simulink library "LibEEPROM_eeprom_example_ORIGINAL"  (Simulink 10.0)
settings: Solver=VariableStepAuto  StartTime=0.0  StopTime=10.0  RelTol=1e-3
undefined symbols (not defined in the file): CRC32_calc_and_EEPROM_Write_ALL, crc32_calc_intern, CRC32_EEPROM_Read, EEPROM_Mirror, EEPROM_Read, IO_Blk_Lib_TTC500, IO_EEPROM_GetStatus, IO_EEPROM_Init, IO_EEPROM_Write, Read_Mirror, Write_Mirror, Write_Mirror_prepare_EEPROM
libraries: simulink x56
(part 3 of 8)

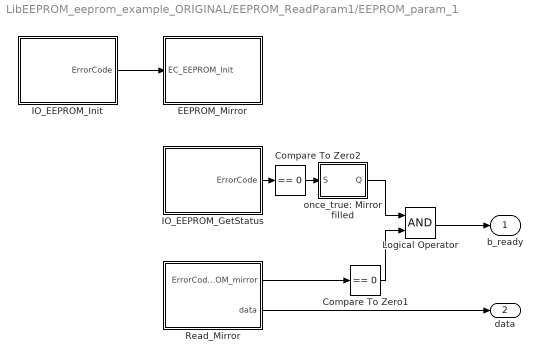
== system LibEEPROM_eeprom_example_ORIGINAL/EEPROM_ReadParam1/EEPROM_param_1 ==
  Compare To Zero1 : simulink/Logic and Bit Operations/Compare To Zero  relop===  OutDataTypeStr=boolean  ZeroCross=off
  Compare To Zero2 : simulink/Logic and Bit Operations/Compare To Zero  relop===  OutDataTypeStr=boolean  ZeroCross=off
  EEPROM_Mirror : Subsystem  LoadFcn=|  mask(EEPROM_Mirror_Code){SampleTime=-1, ttlib=IO_Blk_Lib_TTC500, ttDescription=EEPROM_Mirror, tt_iolib_version=0.21, offset=0, length=65536}
      | try
      | %
      | %Upgrade Information - standard BEGIN
      | new_color = 'blue';
      | new_ver = '0.21';
      | act_ver = get_param(gcb,'tt_iolib_version');
      | if not(strcmp(act_ver,new_ver))
      |     disp(['Upgrade block: ',gcb,char(10),'       Version: ',act_ver,' -> ',new_ver]);
      |     %switch - case for specific upgrade information e.g. additional parameter required 
      |     %Change appearance and version information
      |     set_param(gcb,'ForegroundColor',new_color);
      |     set_param(gcb,'tt_iolib_version',new_ver);
      | end
      | %Upgrade Information - standard END
      | catch
      | %Standard catch section BEGIN 
      | disp(' ');
      | disp('------------------------------------------------------------');
      | disp('An error occurred in a callback of the TTC580-BlockLib.');
      | disp(['Please check the parameters in the mask of ',gcb]);
      | disp('If you do not encounter any violations, then please '); 
      | disp('copy the following lines and report this to support@ttcontrol.com ');
      | disp('<< begin of error message dump >>');
      | disp(['Version of TTC580-BlockLib: ', get_param(gcb,'tt_iolib_version')]);
      | disp(get_param(gcb,'ttDescription'));
      | disp(gcb);
      | x=lasterror;disp(x.message);
      | disp(get_param(gcb,'MaskValues'));
      | disp(version);
      | disp(computer);
      | disp('<< end of error message dump >>');
      | disp('------------------------------------------------------------');
      | disp(' ');
      | %Standard catch section END
      | end
      mask help:
      | Read all data from the EEPROM and mirror this onto RAM.
      | The ErrorCode of IO_EEPROM_Init - block must be connected to the input of EEPROM_Mirror.
      | After calling EEPROM_Mirror the global variable EEPROM_mirror is filled and
      | the global variable ErrorCode_EEPROM_mirror contains the returns of IO_EEPROM_Init() and IO_EEPROM_Read().
      mask init:
      | %
      settings: CopyFcn=%deleted
      mask Help: web(which('IO_EEPROM.h'))
      mask Callback offset: %
      mask Callback length: %
  IO_EEPROM_GetStatus : Subsystem  LoadFcn=|  mask(IO_EEPROM_GetStatus_Code){SampleTime=-1, ttlib=IO_Blk_Lib_TTC500, ttDescription=IO_EEPROM_GetStatus, tt_iolib_version=0.19}
      | try
      | %
      | %Upgrade Information - standard BEGIN
      | new_color = 'blue';
      | new_ver = '0.19';
      | act_ver = get_param(gcb,'tt_iolib_version');
      | if not(strcmp(act_ver,new_ver))
      |     disp(['Upgrade block: ',gcb,char(10),'       Version: ',act_ver,' -> ',new_ver]);
      |     %switch - case for specific upgrade information e.g. additional parameter required 
      |     %Change appearance and version information
      |     set_param(gcb,'ForegroundColor',new_color);
      |     set_param(gcb,'tt_iolib_version',new_ver);
      | end
      | %Upgrade Information - standard END
      | catch
      | %Standard catch section BEGIN 
      | disp(' ');
      | disp('------------------------------------------------------------');
      | disp('An error occurred in a callback of the TTC580-BlockLib.');
      | disp(['Please check the parameters in the mask of ',gcb]);
      | disp('If you do not encounter any violations, then please '); 
      | disp('copy the following lines and report this to support@ttcontrol.com ');
      | disp('<< begin of error message dump >>');
      | disp(['Version of TTC580-BlockLib: ', get_param(gcb,'tt_iolib_version')]);
      | disp(get_param(gcb,'ttDescription'));
      | disp(gcb);
      | x=lasterror;disp(x.message);
      | disp(get_param(gcb,'MaskValues'));
      | disp(version);
      | disp(computer);
      | disp('<< end of error message dump >>');
      | disp('------------------------------------------------------------');
      | disp(' ');
      | %Standard catch section END
      | end
      mask help: Returns the status of the EEPROM driver.
      mask init:
      | %
      settings: CopyFcn=%deleted
      mask Help: web(which('IO_EEPROM.h'))
  IO_EEPROM_Init : Subsystem  LoadFcn=|  mask(IO_EEPROM_Init_Code){SampleTime=-1, ttlib=IO_Blk_Lib_TTC500, ttDescription=IO_EEPROM_Init, tt_iolib_version=0.19}
      | try
      | %
      | %Upgrade Information - standard BEGIN
      | new_color = 'blue';
      | new_ver = '0.19';
      | act_ver = get_param(gcb,'tt_iolib_version');
      | if not(strcmp(act_ver,new_ver))
      |     disp(['Upgrade block: ',gcb,char(10),'       Version: ',act_ver,' -> ',new_ver]);
      |     %switch - case for specific upgrade information e.g. additional parameter required 
      |     %Change appearance and version information
      |     set_param(gcb,'ForegroundColor',new_color);
      |     set_param(gcb,'tt_iolib_version',new_ver);
      | end
      | %Upgrade Information - standard END
      | catch
      | %Standard catch section BEGIN 
      | disp(' ');
      | disp('------------------------------------------------------------');
      | disp('An error occurred in a callback of the TTC580-BlockLib.');
      | disp(['Please check the parameters in the mask of ',gcb]);
      | disp('If you do not encounter any violations, then please '); 
      | disp('copy the following lines and report this to support@ttcontrol.com ');
      | disp('<< begin of error message dump >>');
      | disp(['Version of TTC580-BlockLib: ', get_param(gcb,'tt_iolib_version')]);
      | disp(get_param(gcb,'ttDescription'));
      | disp(gcb);
      | x=lasterror;disp(x.message);
      | disp(get_param(gcb,'MaskValues'));
      | disp(version);
      | disp(computer);
      | disp('<< end of error message dump >>');
      | disp('------------------------------------------------------------');
      | disp(' ');
      | %Standard catch section END
      | end
      mask help: Initialization of the EEPROM driver.
      mask init:
      | %
      settings: CopyFcn=%deleted
      mask Help: web(which('IO_EEPROM.h'))
  Logical Operator : Logic  AllPortsSameDT=off  OutDataTypeStr=boolean
  Read_Mirror : Subsystem  LoadFcn=|  mask(Read_Mirror_Code){SampleTime=-1, ttlib=IO_Blk_Lib_TTC500, ttDescription=Read_Mirror, tt_iolib_version=0.19, offset=offset, length=length}
      | try
      | %
      | %Upgrade Information - standard BEGIN
      | new_color = 'blue';
      | new_ver = '0.19';
      | act_ver = get_param(gcb,'tt_iolib_version');
      | if not(strcmp(act_ver,new_ver))
      |     disp(['Upgrade block: ',gcb,char(10),'       Version: ',act_ver,' -> ',new_ver]);
      |     %switch - case for specific upgrade information e.g. additional parameter required 
      |     %Change appearance and version information
      |     set_param(gcb,'ForegroundColor',new_color);
      |     set_param(gcb,'tt_iolib_version',new_ver);
      | end
      | %Upgrade Information - standard END
      | catch
      | %Standard catch section BEGIN 
      | disp(' ');
      | disp('------------------------------------------------------------');
      | disp('An error occurred in a callback of the TTC580-BlockLib.');
      | disp(['Please check the parameters in the mask of ',gcb]);
      | disp('If you do not encounter any violations, then please '); 
      | disp('copy the following lines and report this to support@ttcontrol.com ');
      | disp('<< begin of error message dump >>');
      | disp(['Version of TTC580-BlockLib: ', get_param(gcb,'tt_iolib_version')]);
      | disp(get_param(gcb,'ttDescription'));
      | disp(gcb);
      | x=lasterror;disp(x.message);
      | disp(get_param(gcb,'MaskValues'));
      | disp(version);
      | disp(computer);
      | disp('<< end of error message dump >>');
      | disp('------------------------------------------------------------');
      | disp(' ');
      | %Standard catch section END
      | end
      mask help:
      | Read data from the mirror of the EEPROM.
      | In case the given data section exceeds given EEPROM boundaries, IO_E_EEPROM_RANGE ErrorCode is returned.
      mask init:
      | %
      settings: CopyFcn=%deleted
      mask Help: web(which('~.h'))
      mask Callback offset: %
      mask Callback length: %
  once_true: Mirror filled : Subsystem  mask(SRFlipFlop){initial_condition=0}
      mask prompts: initial_condition "Initial condition (state of Q):"
      mask help: S-R Flip-Flop Block
      mask Help:
      | The S-R flip-flop also known as a set-reset flip-flop. This implementation
      | is modeled after an S-R flip-flop constructed using NOR gates. The
      | truth table for this block is:
      | <pre>
      |  S  R   Q  !Q
      |  ----------------
      |  1  0   1  0
      |  0  0   1  0  (after S == 1, R == 0)
      |  0  1   0  1
      |  0  0   0  1  (after S == 0, R == 1)
      |  1  1   0  0
      | </pre>
      | 
      | In an S-R flip-flop that is implemented with NOR gates, when a 1 is
      | applied to both the set and reset inputs, both outputs go to 0. Technically,
      | this state is undefined and is usually avoided. Note, if the flip-flop is
      | implemented with NAND gates, when a 0 is applied to both inputs, both outputs
      | go to 0 and when a 1 is applied to both inputs, the output depends on
      | the previous state of the flip-flop (previous value of Q).
  b_ready : Outport  VectorParamsAs1DForOutWhenUnconnected=off
  data : Outport  Port=2  OutDataTypeStr=EEPROM_type  VectorParamsAs1DForOutWhenUnconnected=off
  wires:
  once_true: Mirror filled/1(Q) -> Logical Operator/1
  Compare To Zero2/1 -> once_true: Mirror filled/1(S)
  Compare To Zero1/1 -> Logical Operator/2
  Logical Operator/1 -> b_ready/1
  IO_EEPROM_GetStatus/1(ErrorCode) -> Compare To Zero2/1
  IO_EEPROM_Init/1(ErrorCode) -> EEPROM_Mirror/1(EC_EEPROM_Init)
  Read_Mirror/1(ErrorCode_EEPROM_mirror) -> Compare To Zero1/1
  Read_Mirror/2(data) -> data/1

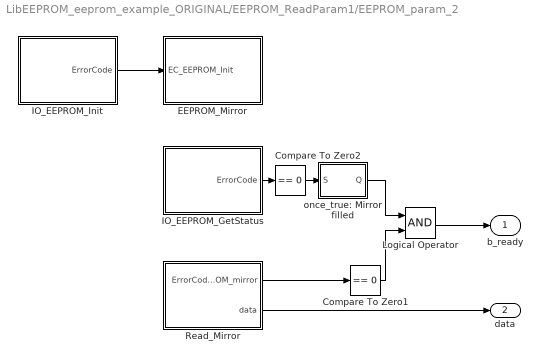
== system LibEEPROM_eeprom_example_ORIGINAL/EEPROM_ReadParam1/EEPROM_param_2 ==
  Compare To Zero1 : simulink/Logic and Bit Operations/Compare To Zero  relop===  OutDataTypeStr=boolean  ZeroCross=off
  Compare To Zero2 : simulink/Logic and Bit Operations/Compare To Zero  relop===  OutDataTypeStr=boolean  ZeroCross=off
  EEPROM_Mirror : Subsystem  LoadFcn=|  mask(EEPROM_Mirror_Code){SampleTime=-1, ttlib=IO_Blk_Lib_TTC500, ttDescription=EEPROM_Mirror, tt_iolib_version=0.21, offset=0, length=65536}
      | try
      | %
      | %Upgrade Information - standard BEGIN
      | new_color = 'blue';
      | new_ver = '0.21';
      | act_ver = get_param(gcb,'tt_iolib_version');
      | if not(strcmp(act_ver,new_ver))
      |     disp(['Upgrade block: ',gcb,char(10),'       Version: ',act_ver,' -> ',new_ver]);
      |     %switch - case for specific upgrade information e.g. additional parameter required 
      |     %Change appearance and version information
      |     set_param(gcb,'ForegroundColor',new_color);
      |     set_param(gcb,'tt_iolib_version',new_ver);
      | end
      | %Upgrade Information - standard END
      | catch
      | %Standard catch section BEGIN 
      | disp(' ');
      | disp('------------------------------------------------------------');
      | disp('An error occurred in a callback of the TTC580-BlockLib.');
      | disp(['Please check the parameters in the mask of ',gcb]);
      | disp('If you do not encounter any violations, then please '); 
      | disp('copy the following lines and report this to support@ttcontrol.com ');
      | disp('<< begin of error message dump >>');
      | disp(['Version of TTC580-BlockLib: ', get_param(gcb,'tt_iolib_version')]);
      | disp(get_param(gcb,'ttDescription'));
      | disp(gcb);
      | x=lasterror;disp(x.message);
      | disp(get_param(gcb,'MaskValues'));
      | disp(version);
      | disp(computer);
      | disp('<< end of error message dump >>');
      | disp('------------------------------------------------------------');
      | disp(' ');
      | %Standard catch section END
      | end
      mask help:
      | Read all data from the EEPROM and mirror this onto RAM.
      | The ErrorCode of IO_EEPROM_Init - block must be connected to the input of EEPROM_Mirror.
      | After calling EEPROM_Mirror the global variable EEPROM_mirror is filled and
      | the global variable ErrorCode_EEPROM_mirror contains the returns of IO_EEPROM_Init() and IO_EEPROM_Read().
      mask init:
      | %
      settings: CopyFcn=%deleted
      mask Help: web(which('IO_EEPROM.h'))
      mask Callback offset: %
      mask Callback length: %
  IO_EEPROM_GetStatus : Subsystem  LoadFcn=|  mask(IO_EEPROM_GetStatus_Code){SampleTime=-1, ttlib=IO_Blk_Lib_TTC500, ttDescription=IO_EEPROM_GetStatus, tt_iolib_version=0.19}
      | try
      | %
      | %Upgrade Information - standard BEGIN
      | new_color = 'blue';
      | new_ver = '0.19';
      | act_ver = get_param(gcb,'tt_iolib_version');
      | if not(strcmp(act_ver,new_ver))
      |     disp(['Upgrade block: ',gcb,char(10),'       Version: ',act_ver,' -> ',new_ver]);
      |     %switch - case for specific upgrade information e.g. additional parameter required 
      |     %Change appearance and version information
      |     set_param(gcb,'ForegroundColor',new_color);
      |     set_param(gcb,'tt_iolib_version',new_ver);
      | end
      | %Upgrade Information - standard END
      | catch
      | %Standard catch section BEGIN 
      | disp(' ');
      | disp('------------------------------------------------------------');
      | disp('An error occurred in a callback of the TTC580-BlockLib.');
      | disp(['Please check the parameters in the mask of ',gcb]);
      | disp('If you do not encounter any violations, then please '); 
      | disp('copy the following lines and report this to support@ttcontrol.com ');
      | disp('<< begin of error message dump >>');
      | disp(['Version of TTC580-BlockLib: ', get_param(gcb,'tt_iolib_version')]);
      | disp(get_param(gcb,'ttDescription'));
      | disp(gcb);
      | x=lasterror;disp(x.message);
      | disp(get_param(gcb,'MaskValues'));
      | disp(version);
      | disp(computer);
      | disp('<< end of error message dump >>');
      | disp('------------------------------------------------------------');
      | disp(' ');
      | %Standard catch section END
      | end
      mask help: Returns the status of the EEPROM driver.
      mask init:
      | %
      settings: CopyFcn=%deleted
      mask Help: web(which('IO_EEPROM.h'))
  IO_EEPROM_Init : Subsystem  LoadFcn=|  mask(IO_EEPROM_Init_Code){SampleTime=-1, ttlib=IO_Blk_Lib_TTC500, ttDescription=IO_EEPROM_Init, tt_iolib_version=0.19}
      | try
      | %
      | %Upgrade Information - standard BEGIN
      | new_color = 'blue';
      | new_ver = '0.19';
      | act_ver = get_param(gcb,'tt_iolib_version');
      | if not(strcmp(act_ver,new_ver))
      |     disp(['Upgrade block: ',gcb,char(10),'       Version: ',act_ver,' -> ',new_ver]);
      |     %switch - case for specific upgrade information e.g. additional parameter required 
      |     %Change appearance and version information
      |     set_param(gcb,'ForegroundColor',new_color);
      |     set_param(gcb,'tt_iolib_version',new_ver);
      | end
      | %Upgrade Information - standard END
      | catch
      | %Standard catch section BEGIN 
      | disp(' ');
      | disp('------------------------------------------------------------');
      | disp('An error occurred in a callback of the TTC580-BlockLib.');
      | disp(['Please check the parameters in the mask of ',gcb]);
      | disp('If you do not encounter any violations, then please '); 
      | disp('copy the following lines and report this to support@ttcontrol.com ');
      | disp('<< begin of error message dump >>');
      | disp(['Version of TTC580-BlockLib: ', get_param(gcb,'tt_iolib_version')]);
      | disp(get_param(gcb,'ttDescription'));
      | disp(gcb);
      | x=lasterror;disp(x.message);
      | disp(get_param(gcb,'MaskValues'));
      | disp(version);
      | disp(computer);
      | disp('<< end of error message dump >>');
      | disp('------------------------------------------------------------');
      | disp(' ');
      | %Standard catch section END
      | end
      mask help: Initialization of the EEPROM driver.
      mask init:
      | %
      settings: CopyFcn=%deleted
      mask Help: web(which('IO_EEPROM.h'))
  Logical Operator : Logic  AllPortsSameDT=off  OutDataTypeStr=boolean
  Read_Mirror : Subsystem  LoadFcn=|  mask(Read_Mirror_Code){SampleTime=-1, ttlib=IO_Blk_Lib_TTC500, ttDescription=Read_Mirror, tt_iolib_version=0.19, offset=offset, length=length}
      | try
      | %
      | %Upgrade Information - standard BEGIN
      | new_color = 'blue';
      | new_ver = '0.19';
      | act_ver = get_param(gcb,'tt_iolib_version');
      | if not(strcmp(act_ver,new_ver))
      |     disp(['Upgrade block: ',gcb,char(10),'       Version: ',act_ver,' -> ',new_ver]);
      |     %switch - case for specific upgrade information e.g. additional parameter required 
      |     %Change appearance and version information
      |     set_param(gcb,'ForegroundColor',new_color);
      |     set_param(gcb,'tt_iolib_version',new_ver);
      | end
      | %Upgrade Information - standard END
      | catch
      | %Standard catch section BEGIN 
      | disp(' ');
      | disp('------------------------------------------------------------');
      | disp('An error occurred in a callback of the TTC580-BlockLib.');
      | disp(['Please check the parameters in the mask of ',gcb]);
      | disp('If you do not encounter any violations, then please '); 
      | disp('copy the following lines and report this to support@ttcontrol.com ');
      | disp('<< begin of error message dump >>');
      | disp(['Version of TTC580-BlockLib: ', get_param(gcb,'tt_iolib_version')]);
      | disp(get_param(gcb,'ttDescription'));
      | disp(gcb);
      | x=lasterror;disp(x.message);
      | disp(get_param(gcb,'MaskValues'));
      | disp(version);
      | disp(computer);
      | disp('<< end of error message dump >>');
      | disp('------------------------------------------------------------');
      | disp(' ');
      | %Standard catch section END
      | end
      mask help:
      | Read data from the mirror of the EEPROM.
      | In case the given data section exceeds given EEPROM boundaries, IO_E_EEPROM_RANGE ErrorCode is returned.
      mask init:
      | %
      settings: CopyFcn=%deleted
      mask Help: web(which('~.h'))
      mask Callback offset: %
      mask Callback length: %
  once_true: Mirror filled : Subsystem  mask(SRFlipFlop){initial_condition=0}
      mask prompts: initial_condition "Initial condition (state of Q):"
      mask help: S-R Flip-Flop Block
      mask Help:
      | The S-R flip-flop also known as a set-reset flip-flop. This implementation
      | is modeled after an S-R flip-flop constructed using NOR gates. The
      | truth table for this block is:
      | <pre>
      |  S  R   Q  !Q
      |  ----------------
      |  1  0   1  0
      |  0  0   1  0  (after S == 1, R == 0)
      |  0  1   0  1
      |  0  0   0  1  (after S == 0, R == 1)
      |  1  1   0  0
      | </pre>
      | 
      | In an S-R flip-flop that is implemented with NOR gates, when a 1 is
      | applied to both the set and reset inputs, both outputs go to 0. Technically,
      | this state is undefined and is usually avoided. Note, if the flip-flop is
      | implemented with NAND gates, when a 0 is applied to both inputs, both outputs
      | go to 0 and when a 1 is applied to both inputs, the output depends on
      | the previous state of the flip-flop (previous value of Q).
  b_ready : Outport  VectorParamsAs1DForOutWhenUnconnected=off
  data : Outport  Port=2  OutDataTypeStr=EEPROM_type  VectorParamsAs1DForOutWhenUnconnected=off
  wires:
  once_true: Mirror filled/1(Q) -> Logical Operator/1
  Compare To Zero2/1 -> once_true: Mirror filled/1(S)
  Compare To Zero1/1 -> Logical Operator/2
  Logical Operator/1 -> b_ready/1
  IO_EEPROM_GetStatus/1(ErrorCode) -> Compare To Zero2/1
  IO_EEPROM_Init/1(ErrorCode) -> EEPROM_Mirror/1(EC_EEPROM_Init)
  Read_Mirror/1(ErrorCode_EEPROM_mirror) -> Compare To Zero1/1
  Read_Mirror/2(data) -> data/1

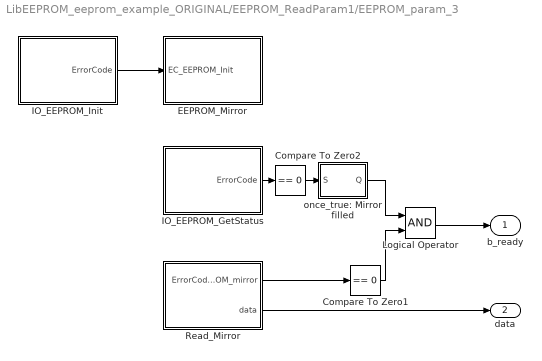
== system LibEEPROM_eeprom_example_ORIGINAL/EEPROM_ReadParam1/EEPROM_param_3 ==
  Compare To Zero1 : simulink/Logic and Bit Operations/Compare To Zero  relop===  OutDataTypeStr=boolean  ZeroCross=off
  Compare To Zero2 : simulink/Logic and Bit Operations/Compare To Zero  relop===  OutDataTypeStr=boolean  ZeroCross=off
  EEPROM_Mirror : Subsystem  LoadFcn=|  mask(EEPROM_Mirror_Code){SampleTime=-1, ttlib=IO_Blk_Lib_TTC500, ttDescription=EEPROM_Mirror, tt_iolib_version=0.21, offset=0, length=65536}
      | try
      | %
      | %Upgrade Information - standard BEGIN
      | new_color = 'blue';
      | new_ver = '0.21';
      | act_ver = get_param(gcb,'tt_iolib_version');
      | if not(strcmp(act_ver,new_ver))
      |     disp(['Upgrade block: ',gcb,char(10),'       Version: ',act_ver,' -> ',new_ver]);
      |     %switch - case for specific upgrade information e.g. additional parameter required 
      |     %Change appearance and version information
      |     set_param(gcb,'ForegroundColor',new_color);
      |     set_param(gcb,'tt_iolib_version',new_ver);
      | end
      | %Upgrade Information - standard END
      | catch
      | %Standard catch section BEGIN 
      | disp(' ');
      | disp('------------------------------------------------------------');
      | disp('An error occurred in a callback of the TTC580-BlockLib.');
      | disp(['Please check the parameters in the mask of ',gcb]);
      | disp('If you do not encounter any violations, then please '); 
      | disp('copy the following lines and report this to support@ttcontrol.com ');
      | disp('<< begin of error message dump >>');
      | disp(['Version of TTC580-BlockLib: ', get_param(gcb,'tt_iolib_version')]);
      | disp(get_param(gcb,'ttDescription'));
      | disp(gcb);
      | x=lasterror;disp(x.message);
      | disp(get_param(gcb,'MaskValues'));
      | disp(version);
      | disp(computer);
      | disp('<< end of error message dump >>');
      | disp('------------------------------------------------------------');
      | disp(' ');
      | %Standard catch section END
      | end
      mask help:
      | Read all data from the EEPROM and mirror this onto RAM.
      | The ErrorCode of IO_EEPROM_Init - block must be connected to the input of EEPROM_Mirror.
      | After calling EEPROM_Mirror the global variable EEPROM_mirror is filled and
      | the global variable ErrorCode_EEPROM_mirror contains the returns of IO_EEPROM_Init() and IO_EEPROM_Read().
      mask init:
      | %
      settings: CopyFcn=%deleted
      mask Help: web(which('IO_EEPROM.h'))
      mask Callback offset: %
      mask Callback length: %
  IO_EEPROM_GetStatus : Subsystem  LoadFcn=|  mask(IO_EEPROM_GetStatus_Code){SampleTime=-1, ttlib=IO_Blk_Lib_TTC500, ttDescription=IO_EEPROM_GetStatus, tt_iolib_version=0.19}
      | try
      | %
      | %Upgrade Information - standard BEGIN
      | new_color = 'blue';
      | new_ver = '0.19';
      | act_ver = get_param(gcb,'tt_iolib_version');
      | if not(strcmp(act_ver,new_ver))
      |     disp(['Upgrade block: ',gcb,char(10),'       Version: ',act_ver,' -> ',new_ver]);
      |     %switch - case for specific upgrade information e.g. additional parameter required 
      |     %Change appearance and version information
      |     set_param(gcb,'ForegroundColor',new_color);
      |     set_param(gcb,'tt_iolib_version',new_ver);
      | end
      | %Upgrade Information - standard END
      | catch
      | %Standard catch section BEGIN 
      | disp(' ');
      | disp('------------------------------------------------------------');
      | disp('An error occurred in a callback of the TTC580-BlockLib.');
      | disp(['Please check the parameters in the mask of ',gcb]);
      | disp('If you do not encounter any violations, then please '); 
      | disp('copy the following lines and report this to support@ttcontrol.com ');
      | disp('<< begin of error message dump >>');
      | disp(['Version of TTC580-BlockLib: ', get_param(gcb,'tt_iolib_version')]);
      | disp(get_param(gcb,'ttDescription'));
      | disp(gcb);
      | x=lasterror;disp(x.message);
      | disp(get_param(gcb,'MaskValues'));
      | disp(version);
      | disp(computer);
      | disp('<< end of error message dump >>');
      | disp('------------------------------------------------------------');
      | disp(' ');
      | %Standard catch section END
      | end
      mask help: Returns the status of the EEPROM driver.
      mask init:
      | %
      settings: CopyFcn=%deleted
      mask Help: web(which('IO_EEPROM.h'))
  IO_EEPROM_Init : Subsystem  LoadFcn=|  mask(IO_EEPROM_Init_Code){SampleTime=-1, ttlib=IO_Blk_Lib_TTC500, ttDescription=IO_EEPROM_Init, tt_iolib_version=0.19}
      | try
      | %
      | %Upgrade Information - standard BEGIN
      | new_color = 'blue';
      | new_ver = '0.19';
      | act_ver = get_param(gcb,'tt_iolib_version');
      | if not(strcmp(act_ver,new_ver))
      |     disp(['Upgrade block: ',gcb,char(10),'       Version: ',act_ver,' -> ',new_ver]);
      |     %switch - case for specific upgrade information e.g. additional parameter required 
      |     %Change appearance and version information
      |     set_param(gcb,'ForegroundColor',new_color);
      |     set_param(gcb,'tt_iolib_version',new_ver);
      | end
      | %Upgrade Information - standard END
      | catch
      | %Standard catch section BEGIN 
      | disp(' ');
      | disp('------------------------------------------------------------');
      | disp('An error occurred in a callback of the TTC580-BlockLib.');
      | disp(['Please check the parameters in the mask of ',gcb]);
      | disp('If you do not encounter any violations, then please '); 
      | disp('copy the following lines and report this to support@ttcontrol.com ');
      | disp('<< begin of error message dump >>');
      | disp(['Version of TTC580-BlockLib: ', get_param(gcb,'tt_iolib_version')]);
      | disp(get_param(gcb,'ttDescription'));
      | disp(gcb);
      | x=lasterror;disp(x.message);
      | disp(get_param(gcb,'MaskValues'));
      | disp(version);
      | disp(computer);
      | disp('<< end of error message dump >>');
      | disp('------------------------------------------------------------');
      | disp(' ');
      | %Standard catch section END
      | end
      mask help: Initialization of the EEPROM driver.
      mask init:
      | %
      settings: CopyFcn=%deleted
      mask Help: web(which('IO_EEPROM.h'))
  Logical Operator : Logic  AllPortsSameDT=off  OutDataTypeStr=boolean
  Read_Mirror : Subsystem  LoadFcn=|  mask(Read_Mirror_Code){SampleTime=-1, ttlib=IO_Blk_Lib_TTC500, ttDescription=Read_Mirror, tt_iolib_version=0.19, offset=offset, length=length}
      | try
      | %
      | %Upgrade Information - standard BEGIN
      | new_color = 'blue';
      | new_ver = '0.19';
      | act_ver = get_param(gcb,'tt_iolib_version');
      | if not(strcmp(act_ver,new_ver))
      |     disp(['Upgrade block: ',gcb,char(10),'       Version: ',act_ver,' -> ',new_ver]);
      |     %switch - case for specific upgrade information e.g. additional parameter required 
      |     %Change appearance and version information
      |     set_param(gcb,'ForegroundColor',new_color);
      |     set_param(gcb,'tt_iolib_version',new_ver);
      | end
      | %Upgrade Information - standard END
      | catch
      | %Standard catch section BEGIN 
      | disp(' ');
      | disp('------------------------------------------------------------');
      | disp('An error occurred in a callback of the TTC580-BlockLib.');
      | disp(['Please check the parameters in the mask of ',gcb]);
      | disp('If you do not encounter any violations, then please '); 
      | disp('copy the following lines and report this to support@ttcontrol.com ');
      | disp('<< begin of error message dump >>');
      | disp(['Version of TTC580-BlockLib: ', get_param(gcb,'tt_iolib_version')]);
      | disp(get_param(gcb,'ttDescription'));
      | disp(gcb);
      | x=lasterror;disp(x.message);
      | disp(get_param(gcb,'MaskValues'));
      | disp(version);
      | disp(computer);
      | disp('<< end of error message dump >>');
      | disp('------------------------------------------------------------');
      | disp(' ');
      | %Standard catch section END
      | end
      mask help:
      | Read data from the mirror of the EEPROM.
      | In case the given data section exceeds given EEPROM boundaries, IO_E_EEPROM_RANGE ErrorCode is returned.
      mask init:
      | %
      settings: CopyFcn=%deleted
      mask Help: web(which('~.h'))
      mask Callback offset: %
      mask Callback length: %
  once_true: Mirror filled : Subsystem  mask(SRFlipFlop){initial_condition=0}
      mask prompts: initial_condition "Initial condition (state of Q):"
      mask help: S-R Flip-Flop Block
      mask Help:
      | The S-R flip-flop also known as a set-reset flip-flop. This implementation
      | is modeled after an S-R flip-flop constructed using NOR gates. The
      | truth table for this block is:
      | <pre>
      |  S  R   Q  !Q
      |  ----------------
      |  1  0   1  0
      |  0  0   1  0  (after S == 1, R == 0)
      |  0  1   0  1
      |  0  0   0  1  (after S == 0, R == 1)
      |  1  1   0  0
      | </pre>
      | 
      | In an S-R flip-flop that is implemented with NOR gates, when a 1 is
      | applied to both the set and reset inputs, both outputs go to 0. Technically,
      | this state is undefined and is usually avoided. Note, if the flip-flop is
      | implemented with NAND gates, when a 0 is applied to both inputs, both outputs
      | go to 0 and when a 1 is applied to both inputs, the output depends on
      | the previous state of the flip-flop (previous value of Q).
  b_ready : Outport  VectorParamsAs1DForOutWhenUnconnected=off
  data : Outport  Port=2  OutDataTypeStr=EEPROM_type  VectorParamsAs1DForOutWhenUnconnected=off
  wires:
  once_true: Mirror filled/1(Q) -> Logical Operator/1
  Compare To Zero2/1 -> once_true: Mirror filled/1(S)
  Compare To Zero1/1 -> Logical Operator/2
  Logical Operator/1 -> b_ready/1
  IO_EEPROM_GetStatus/1(ErrorCode) -> Compare To Zero2/1
  IO_EEPROM_Init/1(ErrorCode) -> EEPROM_Mirror/1(EC_EEPROM_Init)
  Read_Mirror/1(ErrorCode_EEPROM_mirror) -> Compare To Zero1/1
  Read_Mirror/2(data) -> data/1

== system LibEEPROM_eeprom_example_ORIGINAL/EEPROM_ReadParam1/EEPROM_param_4 ==
  Compare To Zero1 : simulink/Logic and Bit Operations/Compare To Zero  relop===  OutDataTypeStr=boolean  ZeroCross=off
  Compare To Zero2 : simulink/Logic and Bit Operations/Compare To Zero  relop===  OutDataTypeStr=boolean  ZeroCross=off
  EEPROM_Mirror : Subsystem  LoadFcn=|  mask(EEPROM_Mirror_Code){SampleTime=-1, ttlib=IO_Blk_Lib_TTC500, ttDescription=EEPROM_Mirror, tt_iolib_version=0.21, offset=0, length=65536}
      | try
      | %
      | %Upgrade Information - standard BEGIN
      | new_color = 'blue';
      | new_ver = '0.21';
      | act_ver = get_param(gcb,'tt_iolib_version');
      | if not(strcmp(act_ver,new_ver))
      |     disp(['Upgrade block: ',gcb,char(10),'       Version: ',act_ver,' -> ',new_ver]);
      |     %switch - case for specific upgrade information e.g. additional parameter required 
      |     %Change appearance and version information
      |     set_param(gcb,'ForegroundColor',new_color);
      |     set_param(gcb,'tt_iolib_version',new_ver);
      | end
      | %Upgrade Information - standard END
      | catch
      | %Standard catch section BEGIN 
      | disp(' ');
      | disp('------------------------------------------------------------');
      | disp('An error occurred in a callback of the TTC580-BlockLib.');
      | disp(['Please check the parameters in the mask of ',gcb]);
      | disp('If you do not encounter any violations, then please '); 
      | disp('copy the following lines and report this to support@ttcontrol.com ');
      | disp('<< begin of error message dump >>');
      | disp(['Version of TTC580-BlockLib: ', get_param(gcb,'tt_iolib_version')]);
      | disp(get_param(gcb,'ttDescription'));
      | disp(gcb);
      | x=lasterror;disp(x.message);
      | disp(get_param(gcb,'MaskValues'));
      | disp(version);
      | disp(computer);
      | disp('<< end of error message dump >>');
      | disp('------------------------------------------------------------');
      | disp(' ');
      | %Standard catch section END
      | end
      mask help:
      | Read all data from the EEPROM and mirror this onto RAM.
      | The ErrorCode of IO_EEPROM_Init - block must be connected to the input of EEPROM_Mirror.
      | After calling EEPROM_Mirror the global variable EEPROM_mirror is filled and
      | the global variable ErrorCode_EEPROM_mirror contains the returns of IO_EEPROM_Init() and IO_EEPROM_Read().
      mask init:
      | %
      settings: CopyFcn=%deleted
      mask Help: web(which('IO_EEPROM.h'))
      mask Callback offset: %
      mask Callback length: %
  IO_EEPROM_GetStatus : Subsystem  LoadFcn=|  mask(IO_EEPROM_GetStatus_Code){SampleTime=-1, ttlib=IO_Blk_Lib_TTC500, ttDescription=IO_EEPROM_GetStatus, tt_iolib_version=0.19}
      | try
      | %
      | %Upgrade Information - standard BEGIN
      | new_color = 'blue';
      | new_ver = '0.19';
      | act_ver = get_param(gcb,'tt_iolib_version');
      | if not(strcmp(act_ver,new_ver))
      |     disp(['Upgrade block: ',gcb,char(10),'       Version: ',act_ver,' -> ',new_ver]);
      |     %switch - case for specific upgrade information e.g. additional parameter required 
      |     %Change appearance and version information
      |     set_param(gcb,'ForegroundColor',new_color);
      |     set_param(gcb,'tt_iolib_version',new_ver);
      | end
      | %Upgrade Information - standard END
      | catch
      | %Standard catch section BEGIN 
      | disp(' ');
      | disp('------------------------------------------------------------');
      | disp('An error occurred in a callback of the TTC580-BlockLib.');
      | disp(['Please check the parameters in the mask of ',gcb]);
      | disp('If you do not encounter any violations, then please '); 
      | disp('copy the following lines and report this to support@ttcontrol.com ');
      | disp('<< begin of error message dump >>');
      | disp(['Version of TTC580-BlockLib: ', get_param(gcb,'tt_iolib_version')]);
      | disp(get_param(gcb,'ttDescription'));
      | disp(gcb);
      | x=lasterror;disp(x.message);
      | disp(get_param(gcb,'MaskValues'));
      | disp(version);
      | disp(computer);
      | disp('<< end of error message dump >>');
      | disp('------------------------------------------------------------');
      | disp(' ');
      | %Standard catch section END
      | end
      mask help: Returns the status of the EEPROM driver.
      mask init:
      | %
      settings: CopyFcn=%deleted
      mask Help: web(which('IO_EEPROM.h'))
  IO_EEPROM_Init : Subsystem  LoadFcn=|  mask(IO_EEPROM_Init_Code){SampleTime=-1, ttlib=IO_Blk_Lib_TTC500, ttDescription=IO_EEPROM_Init, tt_iolib_version=0.19}
      | try
      | %
      | %Upgrade Information - standard BEGIN
      | new_color = 'blue';
      | new_ver = '0.19';
      | act_ver = get_param(gcb,'tt_iolib_version');
      | if not(strcmp(act_ver,new_ver))
      |     disp(['Upgrade block: ',gcb,char(10),'       Version: ',act_ver,' -> ',new_ver]);
      |     %switch - case for specific upgrade information e.g. additional parameter required 
      |     %Change appearance and version information
      |     set_param(gcb,'ForegroundColor',new_color);
      |     set_param(gcb,'tt_iolib_version',new_ver);
      | end
      | %Upgrade Information - standard END
      | catch
      | %Standard catch section BEGIN 
      | disp(' ');
      | disp('------------------------------------------------------------');
      | disp('An error occurred in a callback of the TTC580-BlockLib.');
      | disp(['Please check the parameters in the mask of ',gcb]);
      | disp('If you do not encounter any violations, then please '); 
      | disp('copy the following lines and report this to support@ttcontrol.com ');
      | disp('<< begin of error message dump >>');
      | disp(['Version of TTC580-BlockLib: ', get_param(gcb,'tt_iolib_version')]);
      | disp(get_param(gcb,'ttDescription'));
      | disp(gcb);
      | x=lasterror;disp(x.message);
      | disp(get_param(gcb,'MaskValues'));
      | disp(version);
      | disp(computer);
      | disp('<< end of error message dump >>');
      | disp('------------------------------------------------------------');
      | disp(' ');
      | %Standard catch section END
      | end
      mask help: Initialization of the EEPROM driver.
      mask init:
      | %
      settings: CopyFcn=%deleted
      mask Help: web(which('IO_EEPROM.h'))
  Logical Operator : Logic  AllPortsSameDT=off  OutDataTypeStr=boolean
  Read_Mirror : Subsystem  LoadFcn=|  mask(Read_Mirror_Code){SampleTime=-1, ttlib=IO_Blk_Lib_TTC500, ttDescription=Read_Mirror, tt_iolib_version=0.19, offset=offset, length=length}
      | try
      | %
      | %Upgrade Information - standard BEGIN
      | new_color = 'blue';
      | new_ver = '0.19';
      | act_ver = get_param(gcb,'tt_iolib_version');
      | if not(strcmp(act_ver,new_ver))
      |     disp(['Upgrade block: ',gcb,char(10),'       Version: ',act_ver,' -> ',new_ver]);
      |     %switch - case for specific upgrade information e.g. additional parameter required 
      |     %Change appearance and version information
      |     set_param(gcb,'ForegroundColor',new_color);
      |     set_param(gcb,'tt_iolib_version',new_ver);
      | end
      | %Upgrade Information - standard END
      | catch
      | %Standard catch section BEGIN 
      | disp(' ');
      | disp('------------------------------------------------------------');
      | disp('An error occurred in a callback of the TTC580-BlockLib.');
      | disp(['Please check the parameters in the mask of ',gcb]);
      | disp('If you do not encounter any violations, then please '); 
      | disp('copy the following lines and report this to support@ttcontrol.com ');
      | disp('<< begin of error message dump >>');
      | disp(['Version of TTC580-BlockLib: ', get_param(gcb,'tt_iolib_version')]);
      | disp(get_param(gcb,'ttDescription'));
      | disp(gcb);
      | x=lasterror;disp(x.message);
      | disp(get_param(gcb,'MaskValues'));
      | disp(version);
      | disp(computer);
      | disp('<< end of error message dump >>');
      | disp('------------------------------------------------------------');
      | disp(' ');
      | %Standard catch section END
      | end
      mask help:
      | Read data from the mirror of the EEPROM.
      | In case the given data section exceeds given EEPROM boundaries, IO_E_EEPROM_RANGE ErrorCode is returned.
      mask init:
      | %
      settings: CopyFcn=%deleted
      mask Help: web(which('~.h'))
      mask Callback offset: %
      mask Callback length: %
  once_true: Mirror filled : Subsystem  mask(SRFlipFlop){initial_condition=0}
      mask prompts: initial_condition "Initial condition (state of Q):"
      mask help: S-R Flip-Flop Block
      mask Help:
      | The S-R flip-flop also known as a set-reset flip-flop. This implementation
      | is modeled after an S-R flip-flop constructed using NOR gates. The
      | truth table for this block is:
      | <pre>
      |  S  R   Q  !Q
      |  ----------------
      |  1  0   1  0
      |  0  0   1  0  (after S == 1, R == 0)
      |  0  1   0  1
      |  0  0   0  1  (after S == 0, R == 1)
      |  1  1   0  0
      | </pre>
      | 
      | In an S-R flip-flop that is implemented with NOR gates, when a 1 is
      | applied to both the set and reset inputs, both outputs go to 0. Technically,
      | this state is undefined and is usually avoided. Note, if the flip-flop is
      | implemented with NAND gates, when a 0 is applied to both inputs, both outputs
      | go to 0 and when a 1 is applied to both inputs, the output depends on
      | the previous state of the flip-flop (previous value of Q).
  b_ready : Outport  VectorParamsAs1DForOutWhenUnconnected=off
  data : Outport  Port=2  OutDataTypeStr=EEPROM_type  VectorParamsAs1DForOutWhenUnconnected=off
  wires:
  once_true: Mirror filled/1(Q) -> Logical Operator/1
  Compare To Zero2/1 -> once_true: Mirror filled/1(S)
  Compare To Zero1/1 -> Logical Operator/2
  Logical Operator/1 -> b_ready/1
  IO_EEPROM_GetStatus/1(ErrorCode) -> Compare To Zero2/1
  IO_EEPROM_Init/1(ErrorCode) -> EEPROM_Mirror/1(EC_EEPROM_Init)
  Read_Mirror/1(ErrorCode_EEPROM_mirror) -> Compare To Zero1/1
  Read_Mirror/2(data) -> data/1
